simulink subsystem "HW14_Wind_Model"  (R2025a)
settings: Solver=VariableStepAuto  StartTime=0.0  StopTime=10.0  RelTol=1e-3
settings Model: Creator=thatf  LastModifiedBy=thatf
settings RTWCC: GPUComputeCapability=3.5

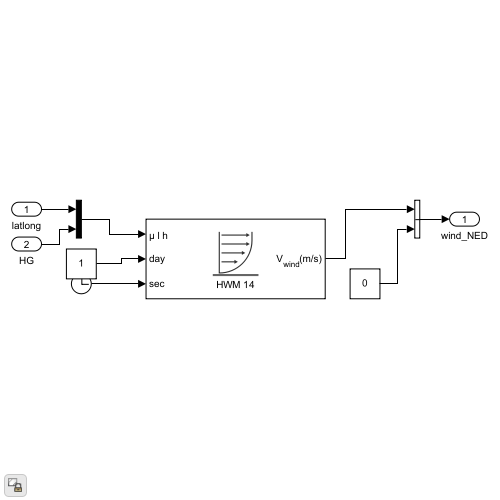
[thumbnail: Simulink's stored preview of the top-level diagram]
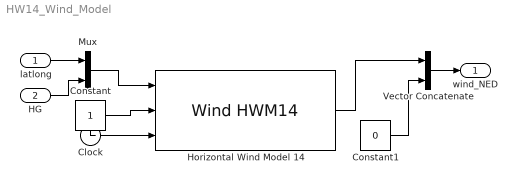
== system HW14_Wind_Model ==
  latlong : Inport
  HG : Inport  Port=2
  Clock : Clock
  Constant : Constant
  Constant1 : Constant  Value=0
  Horizontal Wind Model 14 : WindHWM14
  Mux : Mux  Inputs=2
  Vector Concatenate : Concatenate
  wind_NED : Outport
  wires:
  Horizontal Wind Model 14/1 -> Vector Concatenate/1
  latlong/1 -> Mux/1
  HG/1 -> Mux/2
  Mux/1 -> Horizontal Wind Model 14/1
  Clock/1 -> Horizontal Wind Model 14/3
  Constant/1 -> Horizontal Wind Model 14/2
  Vector Concatenate/1 -> wind_NED/1
  Constant1/1 -> Vector Concatenate/2
